simulink model "subtask2_22_110107589"  (R2022b)
settings: Solver=FixedStepDiscrete  StartTime=0.0  StopTime=(70+1)*8-1  RelTol=1e-3
libraries: dspstat3 x1
settings Model: LastModifiedBy=gowrav -local

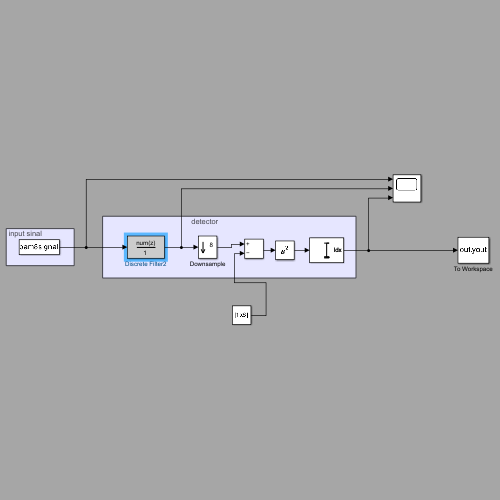
[thumbnail: Simulink's stored preview of the top-level diagram]
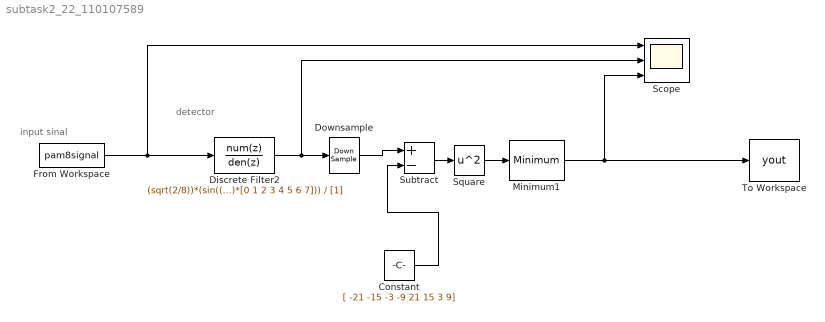
== system subtask2_22_110107589 ==
  note: input sinal
  note: detector
  Constant : Constant  Value=[ -21 -15 -3 -9 21 15 3 9]
  Discrete Filter2 : DiscreteFilter  Numerator=(sqrt(2/8))*(sin((pi/8)*[0 1 2 3 4 5 6 7]))  Denominator=[1]  SampleTime=1
  Downsample : DownSample  N=8  RateOptions=Allow multirate processing
  From Workspace : FromWorkspace  VariableName=pam8signal  SampleTime=1
  Minimum1 : dspstat3/Minimum  operation=minimum  fcn=Index  indexBase=Zero  operateOver=Each column  Dimension=1  InputProcessing=Columns as channels (frame based)  reset=None  roiEnable=off  roiType=Rectangles  roiPortion=Entire ROI  roiOutput=Individual statistics for each ROI  roiFlag=off  roundingMode=Floor  overflowMode=off
  Scope : Scope  NumInputPorts=3
  Square : Math  Operator=square
  Subtract : Sum  Inputs=+-
  To Workspace : ToWorkspace  VariableName=yout  SaveFormat=Timeseries  SampleTime=-1
      settings: Save2DSignal=2-D array (concatenate along first dimension)
  wires:
  Discrete Filter2/1 -> Scope/2, Downsample/1
  From Workspace/1 -> Scope/1, Discrete Filter2/1
  Constant/1 -> Subtract/2
  Subtract/1 -> Square/1
  Minimum1/1 -> To Workspace/1, Scope/3
  Downsample/1 -> Subtract/1
  Square/1 -> Minimum1/1
